simulink model "data_collection"  (R2024a)
settings: Solver=FixedStepAuto  StartTime=0.0  StopTime=inf  FixedStep=0.01  RelTol=1e-3
values from neighbouring files (symbols this model uses):
  omega_max = Simulink.Parameter(425.47)    [katech_automation.m]
  wind_type_toggle = 2    [katech_automation.m]    (also in katech_automation_HILS.m)
  window_size_ = Simulink.Parameter(100)    [katech_automation.m]    (also in katech_automation_HILS.m)
undefined symbols (not defined in the file or in its folder): rad, s, X, Y, Z
libraries: robotlib x28, simulink x14, aerolibconvert2 x2, sharedtransform x1, simulink_extras x1, eeGeneralControl x1
(part 1 of 2)
settings Model: Creator=hmcl  LastModifiedBy=hmcl
settings OptimizationCC: EnhancedBackFolding=on  PassReuseOutputArgsAs=Individual arguments  ZeroExternalMemoryAtStartup=off  ZeroInternalMemoryAtStartup=off  MaxStackSize=64  OptimizeBlockOrder=speed  DifferentSizesBufferReuse=on  OptimizationCustomize=off  EfficientTunableParamExpr=on
settings DebuggingCC: ParameterTunabilityLossMsg=error
settings HardwareCC: ProdBitPerPointer=32  ProdBitPerSizeT=32  ProdBitPerPtrDiffT=32  ProdLargestAtomicFloat=None  ProdIntDivRoundTo=Undefined  ProdEndianess=Unspecified  ProdWordSize=32  ProdHWDeviceType=Generic->Unspecified (assume 32-bit Generic)
settings RTWCC: Description=Embedded Coder  SystemTargetFile=ert.tlc  HardwareBoard=Robot Operating System (ROS)  TLCOptions="-aInlineSetEventsForThisBaseRateFcn=TLC_FALSE -aSuppressMultiTaskScheduler=TLC_FALSE  -aRateBasedStepFcn=0"  TemplateMakefile=ert_default_tmf  Toolchain=Catkin  TargetLang=C++  GPUComputeCapability=3.5
settings CodeAppCC: ForceParamTrailComments=on  IgnoreCustomStorageClasses=off  OperatorAnnotations=on  SimulinkDataObjDesc=on  SFDataObjDesc=on  InsertBlockDesc=on

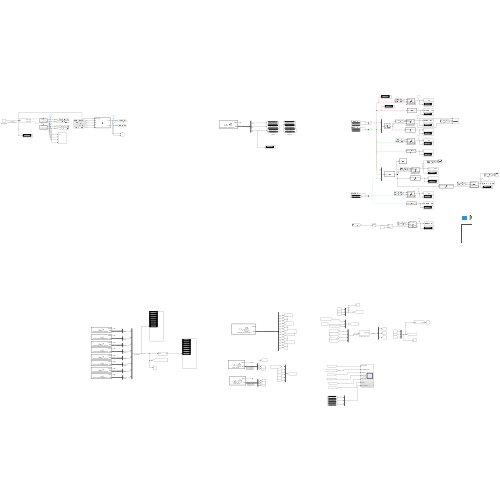
[thumbnail: Simulink's stored preview of the top-level diagram]
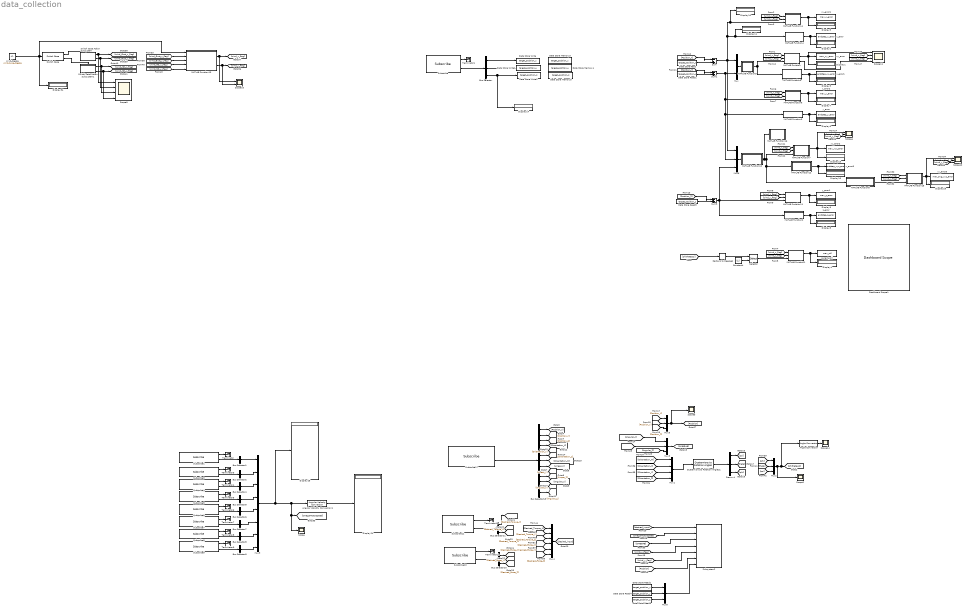
== system data_collection ==
  Angle Conversion : aerolibconvert2/Angle Conversion  IU=rad  OU=deg
  Angular Velocity Conversion1 : aerolibconvert2/Angular Velocity Conversion  IU=rad/s  OU=rpm
  Bus Selector : BusSelector  OutputSignals=Pose.Position.X,Pose.Position.Y,Pose.Position.Z
  Bus Selector{1..2,4..9} (8 alike) : BusSelector  OutputSignals=Data
  Bus Selector10 : BusSelector  OutputSignals=X,Y,Z
  Bus Selector11 : BusSelector  OutputSignals=X,Y,Z
  Bus Selector18 : BusSelector  OutputSignals=Pose.Pose.Position.X,Pose.Pose.Position.Y,Pose.Pose.Position.Z,Pose.Pose.Orientation.X,Pose.Pose.Orientation.Y,Pose.Pose.Orientation.Z,Pose.Pose.Orientation.W,Twist.Twist.Linear.X,Twist.Twist.Linear.Y,Twist.Twist.Linear.Z,Twist.Twist.Angular.X,Twist.Twist.Angular.Y,Twist.Twist.Angular.Z
  Constant4 : Constant  Value=[1]
  Dashboard Scope1 : DashboardScope
  Data Store Memory3 : DataStoreMemory  DataStoreName=target_position_x  ReadBeforeWriteMsg=warning  WriteAfterWriteMsg=warning  WriteAfterReadMsg=warning  ShowAdditionalParam=off
  Data Store Memory4 : DataStoreMemory  DataStoreName=target_position_y  ReadBeforeWriteMsg=warning  WriteAfterWriteMsg=warning  WriteAfterReadMsg=warning  ShowAdditionalParam=off
  Data Store Memory5 : DataStoreMemory  DataStoreName=target_position_z  ReadBeforeWriteMsg=warning  WriteAfterWriteMsg=warning  WriteAfterReadMsg=warning  ShowAdditionalParam=off
  Data Store Read : DataStoreRead  DataStoreName=target_position_x  IndexOptions=Index vector (dialog)  Indices=1  OutputSizes=1
  Data Store Read1 : DataStoreRead  DataStoreName=target_position_y  IndexOptions=Index vector (dialog)  Indices=1  OutputSizes=1
  Data Store Read2 : DataStoreRead  DataStoreName=target_position_x  IndexOptions=Index vector (dialog)  Indices=1  OutputSizes=1
  Data Store Read3 : DataStoreRead  DataStoreName=target_position_z  IndexOptions=Index vector (dialog)  Indices=1  OutputSizes=1
  Data Store Read4 : DataStoreRead  DataStoreName=target_position_y  IndexOptions=Index vector (dialog)  Indices=1  OutputSizes=1
  Data Store Read5 : DataStoreRead  DataStoreName=target_position_z  IndexOptions=Index vector (dialog)  Indices=1  OutputSizes=1
  Data Store Write : DataStoreWrite  DataStoreName=target_position_x  IndexOptions=Index vector (dialog)  Indices=1  OutputSizes=1
  Data Store Write1 : DataStoreWrite  DataStoreName=target_position_y  IndexOptions=Index vector (dialog)  Indices=1  OutputSizes=1
  Data Store Write2 : DataStoreWrite  DataStoreName=target_position_z  IndexOptions=Index vector (dialog)  Indices=1  OutputSizes=1
  Demux4 : Demux  Outputs=3
  Display{1..11,14..16,24..25,29,34} (18 alike) : Display
  MATLAB Function : MATLAB Function  TreatAsAtomicUnit=on
  MATLAB Function1 : MATLAB Function  TreatAsAtomicUnit=on
  MATLAB Function10 : MATLAB Function  TreatAsAtomicUnit=on
  MATLAB Function11 : MATLAB Function  TreatAsAtomicUnit=on
  MATLAB Function12 : MATLAB Function  TreatAsAtomicUnit=on
  MATLAB Function13 : MATLAB Function  TreatAsAtomicUnit=on
  MATLAB Function14 : MATLAB Function  TreatAsAtomicUnit=on
  MATLAB Function15 : MATLAB Function  TreatAsAtomicUnit=on
  MATLAB Function16 : MATLAB Function  TreatAsAtomicUnit=on
  MATLAB Function2 : MATLAB Function  TreatAsAtomicUnit=on
  MATLAB Function3 : MATLAB Function  TreatAsAtomicUnit=on
  MATLAB Function4 : MATLAB Function  TreatAsAtomicUnit=on
  MATLAB Function5 : MATLAB Function  TreatAsAtomicUnit=on
  MATLAB Function6 : MATLAB Function  TreatAsAtomicUnit=on
  MATLAB Function7 : MATLAB Function  TreatAsAtomicUnit=on
  MATLAB Function8 : MATLAB Function  InitFcn=|  TreatAsAtomicUnit=on
      | % 이 코드는 시뮬레이션이 시작되기 직전에 실행됩니다.
      | 
      | % 1. 'window_size_'가 Base Workspace에 '존재하지 않는지' 확인합니다.
      | if ~evalin('base', 'exist(''window_size_'', ''var'')')
      | 
      |     % 존재하지 않으면 (스크립트에서 설정을 잊었으면), 기본값으로 생성합니다.
      |     disp('[InitFcn] "window_size_"를 찾을 수 없습니다. 기본값(100)으로 설정합니다.');
      |     window_size_ = Simulink.Parameter(100);
      | 
      |     % Simulink가 찾을 수 있도록 Base Workspace에 변수를 할당합니다.
      |     assignin('base', 'window_size_', window_size_);
      | end
      | 
      | 
      | try
      |     % 현재 실행 중인 Simulink 모델(.slx)이 저장된 폴더의 '전체 경로'를 찾습니다.
      |     current_model_folder = fileparts(which(bdroot));
      |     
      |     % 'octo_model' 폴더의 '전체 경로'를 생성합니다.
      |     % (Simulink 파일과 'octo_model' 폴더가 같은 디렉터리에 있다고 가정)
      |     path_to_add = fullfile(current_model_folder, 'octo_model');
      |     
      |     % MATLAB 경로에 해당 폴더가 없으면 추가합니다.
      |     if ~contains(path, path_to_add)
      |         disp(['[InitFcn] 함수 경로를 추가합니다: ' path_to_add]);
      |         addpath(path_to_add);
      |     else
      |         disp('[InitFcn] 함수 경로가 이미 설정되어 있습니다.');
      |     end
      | catch ME_path
      |     warndlg(['[InitFcn] 경로 설정 중 심각한 오류 발생: ' ME_path.message], 'InitFcn Error');
      |     return; % 경로 설정 실패 시 중단
      | end
  MATLAB Function9 : MATLAB Function  TreatAsAtomicUnit=on
  Mux : Mux  Inputs=2
  Mux1 : Mux
  Mux{2..3,5..6,8} (5 alike) : Mux  Inputs=3
  Mux4 : Mux  Inputs=6
  Mux9 : Mux  Inputs=8
  Quaternions to Rotation Angles1 : sharedtransform/Quaternions to Rotation Angles  rotationOrder=ZYX  aMode=aMode
  Radians to Degrees : simulink_extras/Transformations/Radians to Degrees
  Scope{,2..3,14} (4 alike) : Scope
  Scope10 : Scope  NumInputPorts=2
  Scope11 : Scope  NumInputPorts=4
  Scope12 : Scope  NumInputPorts=3
  Scope4 : Scope  NumInputPorts=3
  Scope9 : Scope  NumInputPorts=4
  Selector : Selector  InputPortWidth=3  IndexOptions=Index vector (port)  Indices=[1 3]  OutputSizes=1
  Subscribe : robotlib/Subscribe  topicSource=Select from ROS network  topic=/mavros/setpoint_position/local  messageType=geometry_msgs/PoseStamped  SampleTime=-1  legacyBusStruct=off  messageQueueLength=1
  Subscribe1 : robotlib/Subscribe  topicSource=Select from ROS network  topic=/my/octocopter3/motor_speed/0  messageType=std_msgs/Float64  SampleTime=-1  legacyBusStruct=off  messageQueueLength=1
  Subscribe10 : robotlib/Subscribe  topicSource=Select from ROS network  topic=/thrust_vector  messageType=geometry_msgs/Vector3  SampleTime=-1  legacyBusStruct=off  messageQueueLength=1
  Subscribe11 : robotlib/Subscribe  topicSource=Select from ROS network  topic=/torque_vector  messageType=geometry_msgs/Vector3  SampleTime=-1  legacyBusStruct=off  messageQueueLength=1
  Subscribe17 : robotlib/Subscribe  topicSource=Select from ROS network  topic=/mavros/local_position/odom  messageType=nav_msgs/Odometry  SampleTime=-1  legacyBusStruct=off  messageQueueLength=1
  Subscribe3 : robotlib/Subscribe  topicSource=Select from ROS network  topic=/my/octocopter3/motor_speed/1  messageType=std_msgs/Float64  SampleTime=-1  legacyBusStruct=off  messageQueueLength=1
  Subscribe4 : robotlib/Subscribe  topicSource=Select from ROS network  topic=/my/octocopter3/motor_speed/2  messageType=std_msgs/Float64  SampleTime=-1  legacyBusStruct=off  messageQueueLength=1
  Subscribe5 : robotlib/Subscribe  topicSource=Select from ROS network  topic=/my/octocopter3/motor_speed/3  messageType=std_msgs/Float64  SampleTime=-1  legacyBusStruct=off  messageQueueLength=1
  Subscribe6 : robotlib/Subscribe  topicSource=Select from ROS network  topic=/my/octocopter3/motor_speed/4  messageType=std_msgs/Float64  SampleTime=-1  legacyBusStruct=off  messageQueueLength=1
  Subscribe7 : robotlib/Subscribe  topicSource=Select from ROS network  topic=/my/octocopter3/motor_speed/5  messageType=std_msgs/Float64  SampleTime=-1  legacyBusStruct=off  messageQueueLength=1
  Subscribe8 : robotlib/Subscribe  topicSource=Select from ROS network  topic=/my/octocopter3/motor_speed/6  messageType=std_msgs/Float64  SampleTime=-1  legacyBusStruct=off  messageQueueLength=1
  Subscribe9 : robotlib/Subscribe  topicSource=Select from ROS network  topic=/my/octocopter3/motor_speed/7  messageType=std_msgs/Float64  SampleTime=-1  legacyBusStruct=off  messageQueueLength=1
  Subsystem2 : Subsystem
  Sum : Sum  Inputs=|-+
  Sum1 : Sum  Inputs=|-+
  Sum3 : Sum  Inputs=|-+
  Switch Case : SwitchCase  CaseConditions={1,2}  ShowDefaultCase=off
  Switch Case Action Subsystem : Subsystem  TreatAsAtomicUnit=on
  Switch Case Action Subsystem1 : Subsystem  TreatAsAtomicUnit=on
  Terminator{,1,3..11} (11 alike) : Terminator
  current_roll : ToWorkspace  VariableName=max_roll  SampleTime=-1
      settings: Save2DSignal=2-D array (concatenate along first dimension)
  wind_toggle : Constant  InitFcn=|  Value=wind_type_toggle
      | % 이 코드는 시뮬레이션이 시작되기 직전에 실행됩니다.
      | 
      | if ~evalin('base', 'exist(''wind_type_toggle'', ''var'')')
      | 
      |     % 존재하지 않으면 (스크립트에서 설정을 잊었으면), 기본값으로 생성합니다.
      |     disp('[InitFcn] "wind_type_toggle"를 찾을 수 없습니다. 기본값(1, Gust)으로 설정합니다.');
      |     wind_type_toggle = Simulink.Parameter(1);
      | 
      |     % Simulink가 찾을 수 있도록 Base Workspace에 변수를 할당합니다.
      |     assignin('base', 'wind_type_toggle', wind_type_toggle);
      | end
  x_error : ToWorkspace  VariableName=endstep_x_error  SampleTime=-1
      settings: Save2DSignal=2-D array (concatenate along first dimension)
  x_error1 : ToWorkspace  VariableName=endstep_xy_error  SampleTime=-1
      settings: Save2DSignal=2-D array (concatenate along first dimension)
  x_error2 : ToWorkspace  VariableName=max_y_error  SampleTime=-1
      settings: Save2DSignal=2-D array (concatenate along first dimension)
  x_error3 : ToWorkspace  VariableName=endstep_xyz_error  SampleTime=-1
      settings: Save2DSignal=2-D array (concatenate along first dimension)
  xy_error : ToWorkspace  VariableName=max_xy_error  SampleTime=-1
      settings: Save2DSignal=2-D array (concatenate along first dimension)
  xy_error1 : ToWorkspace  VariableName=max_x_error  SampleTime=-1
      settings: Save2DSignal=2-D array (concatenate along first dimension)
  xy_error2 : ToWorkspace  VariableName=max_xyz_error  SampleTime=-1
      settings: Save2DSignal=2-D array (concatenate along first dimension)
  xy_error3 : ToWorkspace  VariableName=max_avg_xyz_error  SampleTime=-1
      settings: Save2DSignal=2-D array (concatenate along first dimension)
  y_error : ToWorkspace  VariableName=endstep_y_error  SampleTime=-1
      settings: Save2DSignal=2-D array (concatenate along first dimension)
  y_error1 : ToWorkspace  VariableName=max_z_error  SampleTime=-1
      settings: Save2DSignal=2-D array (concatenate along first dimension)
  z_error : ToWorkspace  VariableName=endstep_z_error  SampleTime=-1
      settings: Save2DSignal=2-D array (concatenate along first dimension)
  wires:
  Bus Selector/3 -> Display14/1, Data Store Write2/1  "<Z>"
  Subscribe/1 -> Terminator1/1
  Bus Selector/2 -> Data Store Write1/1  "<Y>"
  Bus Selector/1 -> Data Store Write/1  "<X>"
  MATLAB Function3/1(y) -> Display6/1, y_error/1
  MATLAB Function2/1(y) -> Display8/1, z_error/1
  MATLAB Function14/1(y) -> Display5/1, xy_error1/1
  MATLAB Function6/1(y) -> Display7/1, x_error2/1
  MATLAB Function/1(y) -> Scope11/1, xy_error/1, Display1/1
  MATLAB Function4/1(y) -> x_error/1, Display2/1
  MATLAB Function11/1(y) -> Display9/1, y_error1/1
  MATLAB Function9/1(y) -> x_error1/1, Display3/1
  Data Store Read/1 -> Sum/2
  [wind_x_flag] -> MATLAB Function14/1(wind_x_flag)
  [wind_x_flag] -> MATLAB Function6/1(wind_x_flag)
  Sum3/1 -> MATLAB Function11/3(u), Mux6/3, MATLAB Function2/1(endstep_z_error)
  [wind_y_flag] -> MATLAB Function/2(wind_y_flag)
  [wind_x_flag] -> MATLAB Function/1(wind_x_flag)
  MATLAB Function5/1(y) -> MATLAB Function9/1(endstep_xy_error), MATLAB Function/3(u)
  [wind_x_flag] -> MATLAB Function11/1(wind_x_flag)
  Data Store Read3/1 -> Sum3/2
  [wind_y_flag] -> MATLAB Function6/2(wind_y_flag)
  Mux/1 -> MATLAB Function5/1(xy_error)
  [wind_y_flag] -> MATLAB Function11/2(wind_y_flag)
  Sum/1 -> Mux6/1, MATLAB Function14/3(u), Display10/1, Display11/1, MATLAB Function4/1(endstep_x_error), Mux/1
  Sum1/1 -> MATLAB Function6/3(u), Mux6/2, MATLAB Function3/1(endstep_y_error), Mux/2
  Data Store Read1/1 -> Sum1/2
  [wind_y_flag] -> MATLAB Function14/2(wind_y_flag)
  MATLAB Function1/1(y) -> Display4/1, current_roll/1
  Constant4/1 -> Selector/2
  [phithetapsi] -> Radians to Degrees/1
  Selector/1 -> MATLAB Function1/3(u)
  [wind_x_flag] -> MATLAB Function1/1(wind_x_flag)
  [wind_y_flag] -> MATLAB Function1/2(wind_y_flag)
  Radians to Degrees/1 -> Selector/1
  Subscribe/2 -> Bus Selector/1
  [Orientation_W] -> Mux1/1  "W"
  Demux4/3 -> [phi]
  Demux4/1 -> [psi]
  Demux4/2 -> [theta]
  [Orientation_Y] -> Mux1/3  "Y"
  Quaternions to Rotation Angles1/1 -> Demux4/1  "radian"
  [Orientation_X] -> Mux1/2  "x"
  [Orientation_Z] -> Mux1/4  "z"
  Mux1/1 -> Quaternions to Rotation Angles1/1  "quertanion"
  [phi] -> Mux2/1
  Mux2/1 -> Scope2/1, Angle Conversion/1, [phithetapsi]
  [psi] -> Mux2/3
  [theta] -> Mux2/2
  [Position_X] -> Sum/1
  [Position_Y] -> Sum1/1
  [Position_Z] -> Sum3/1
  [Angular_X] -> Mux3/1
  [Angular_Y] -> Mux3/2
  [Angular_Z] -> Mux3/3
  Mux3/1 -> [OMEGAB]
  [OMEGAB] -> Subsystem2/3(OMEGAB)
  [desired_input] -> Subsystem2/1(desired_input)
  [omegaMotorSpeed] -> Subsystem2/2(omegaMotorSpeed)
  Bus Selector8/1 -> Mux9/7  "<Data>"
  Subscribe1/1 -> Terminator/1
  Subscribe8/2 -> Bus Selector8/1
  Subscribe3/1 -> Terminator3/1
  Subscribe3/2 -> Bus Selector2/1
  Subscribe4/2 -> Bus Selector4/1
  Bus Selector4/1 -> Mux9/3  "<Data>"
  Angular Velocity Conversion1/1 -> Display24/1
  Subscribe6/2 -> Bus Selector6/1
  Subscribe4/1 -> Terminator4/1
  Mux9/1 -> Display25/1, Angular Velocity Conversion1/1, Scope/1, [omegaMotorSpeed]  "motorSpeed"
  Subscribe6/1 -> Terminator6/1
  Subscribe9/2 -> Bus Selector9/1
  Bus Selector6/1 -> Mux9/5  "<Data>"
  Subscribe5/2 -> Bus Selector5/1
  Bus Selector9/1 -> Mux9/8  "<Data>"
  Subscribe5/1 -> Terminator5/1
  Subscribe7/1 -> Terminator7/1
  Bus Selector1/1 -> Mux9/1  "<Data>"
  Subscribe1/2 -> Bus Selector1/1
  Subscribe7/2 -> Bus Selector7/1
  Subscribe9/1 -> Terminator9/1
  Subscribe8/1 -> Terminator8/1
  Bus Selector2/1 -> Mux9/2  "<Data>"
  Bus Selector5/1 -> Mux9/4  "<Data>"
  Bus Selector7/1 -> Mux9/6  "<Data>"
  [Desired_Force_X] -> Mux4/4
  [Desired_Torque_Y] -> Mux4/2
  Bus Selector11/3 -> [Desired_Torque_Z]  "<Z>"
  [Desired_Torque_X] -> Mux4/1
  Subscribe10/1 -> Terminator11/1
  Subscribe11/2 -> Bus Selector11/1  "Desired_Torque_X Desired_Torque_Y Desired_Torque_Z"
  [Desired_Torque_Z] -> Mux4/3
  [Desired_Force_Y] -> Mux4/5
  [Desired_Force_Z] -> Mux4/6
  Subscribe11/1 -> Terminator10/1
  Bus Selector10/3 -> [Desired_Force_Z]  "<Z>"
  Bus Selector10/2 -> [Desired_Force_Y]  "<Y>"
  Subscribe10/2 -> Bus Selector10/1  "Desired_Force_X Desired_Force_Y Desired_Force_Z"
  Bus Selector11/1 -> [Desired_Torque_X]  "<X>"
  Bus Selector11/2 -> [Desired_Torque_Y]  "<Y>"
  Bus Selector10/1 -> [Desired_Force_X]  "<X>"
  Mux4/1 -> [desired_input]
  [wind_x_flag] -> Subsystem2/4(wind_x_flag)
  [wind_y_flag] -> Subsystem2/5(wind_y_flag)
  [Position_X] -> Mux5/1
  [Position_Y] -> Mux5/2
  [Position_Z] -> Mux5/3
  Mux5/1 -> Scope3/1, [Position]
  Mux6/1 -> MATLAB Function10/1(xyz_error)
  [wind_x_flag] -> MATLAB Function7/1(wind_x_flag)
  [wind_y_flag] -> MATLAB Function7/2(wind_y_flag)
  MATLAB Function10/1(y) -> MATLAB Function16/1(u), MATLAB Function7/3(u), MATLAB Function8/1(xyz_error), MATLAB Function12/1(endstep_xyz_error)
  MATLAB Function7/1(y) -> Scope4/1, Display15/1, xy_error2/1
  MATLAB Function12/1(y) -> x_error3/1, Display16/1
  [wind_x_flag] -> Scope4/2
  [wind_y_flag] -> Scope4/3
  Switch Case/1 -> Switch Case Action Subsystem/Action
  Switch Case/2 -> Switch Case Action Subsystem1/Action
  Switch Case Action Subsystem1/1(Out1) -> Scope9/3, [wind_ND_x_flag]
  wind_toggle/1 -> Switch Case/1, MATLAB Function13/1(wind_toggle), Display34/1  "1 : Gust 2 : Normal Distribution"
  Switch Case Action Subsystem/1(Out2) -> Scope9/1, [wind_Gust_x_flag]
  Switch Case Action Subsystem/2(Output) -> Scope9/2, [wind_Gust_y_flag]
  MATLAB Function13/1(x_flag) -> Scope10/1, [wind_x_flag]
  MATLAB Function13/2(y_flag) -> Scope10/2, [wind_y_flag]
  [wind_Gust_y_flag] -> MATLAB Function13/3(a2)
  [wind_Gust_x_flag] -> MATLAB Function13/2(a1)
  [wind_ND_x_flag] -> MATLAB Function13/4(a3)
  [wind_ND_y_flag] -> MATLAB Function13/5(a4)
  Switch Case Action Subsystem1/2(Out2) -> Scope9/4, [wind_ND_y_flag]
  [wind_x_flag] -> Scope11/2
  [wind_y_flag] -> Scope11/3
  MATLAB Function/2(toggle_swtich) -> Scope11/4
  Subscribe17/2 -> Bus Selector18/1
  Bus Selector18/1 -> [Position_X]  "<X>"
  Bus Selector18/2 -> [Position_Y]  "<Y>"
  Bus Selector18/3 -> [Position_Z]  "<Z>"
  Bus Selector18/4 -> [Orientation_X]  "<X>"
  Bus Selector18/5 -> [Orientation_Y]  "<Y>"
  Bus Selector18/6 -> [Orientation_Z]  "<Z>"
  Bus Selector18/7 -> [Orientation_W]  "<W>"
  Bus Selector18/8 -> [Linear_X]  "<X>"
  Bus Selector18/9 -> [Linear_Y]  "<Y>"
  Bus Selector18/10 -> [Linear_Z]  "<Z>"
  Bus Selector18/11 -> [Angular_X]  "<X>"
  Bus Selector18/12 -> [Angular_Y]  "<Y>"
  Bus Selector18/13 -> [Angular_Z]  "<Z>"
  [Position] -> Subsystem2/6(Position)
  MATLAB Function8/1(avg_array_xyz_error) -> MATLAB Function15/3(u)
  [wind_x_flag] -> MATLAB Function15/1(wind_x_flag)
  [wind_y_flag] -> MATLAB Function15/2(wind_y_flag)
  [wind_y_flag] -> Scope12/3
  [wind_x_flag] -> Scope12/2
  MATLAB Function15/1(y) -> Display29/1, Scope12/1, xy_error3/1
  Angle Conversion/1 -> Scope14/1
  Data Store Read5/1 -> Mux8/3
  Data Store Read4/1 -> Mux8/2
  Data Store Read2/1 -> Mux8/1
  Mux8/1 -> Subsystem2/7(Target Position)

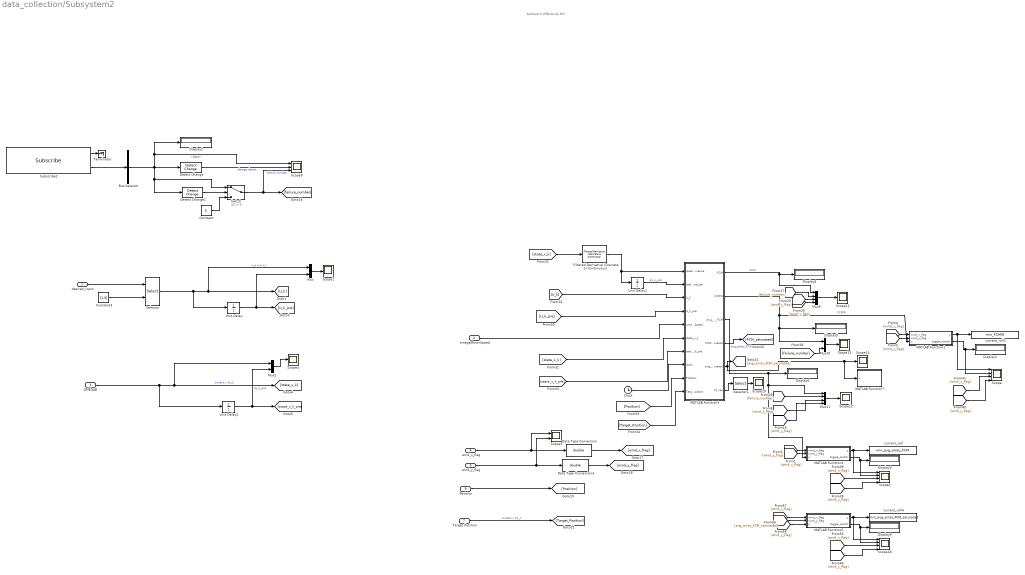
== system data_collection/Subsystem2 ==
  note: backward difference fcm
  desired_input : Inport
  omegaMotorSpeed : Inport  Port=2
  OMEGAB : Inport  Port=3
  wind_x_flag : Inport  Port=4
  wind_y_flag : Inport  Port=5
  Position : Inport  Port=6
  Target Position : Inport  Port=7
  Bus Selector : BusSelector  OutputSignals=Data
  Clock : Clock
  Constant : Constant  Value=0
  Constant4 : Constant  Value=[1:3]
  Data Type Conversion : DataTypeConversion  OutDataTypeStr=double  SaturateOnIntegerOverflow=off  RndMeth=Floor
  Data Type Conversion1 : DataTypeConversion  OutDataTypeStr=double  SaturateOnIntegerOverflow=off  RndMeth=Floor
  Detect Change : simulink/Logic and Bit Operations/Detect Change  vinit=0  OutDataTypeStr=boolean
  Detect Change1 : simulink/Logic and Bit Operations/Detect Change  vinit=0  OutDataTypeStr=boolean
  Display{1..6,9} (7 alike) : Display
  Filtered Derivative (Discrete or Continuous) : eeGeneralControl/Filtered Derivative (Discrete or Continuous)  K=1  T=0.1  B=inf  A=-inf  minRatio=10  init_option=Inherited from block input  x0=0  Ts=-1
      settings: LibrarySourceBlock=|
      | ee_sl_lib/General Control/Filtered Derivative
      | (Discrete or Continuous)
  MATLAB Function2 : MATLAB Function  TreatAsAtomicUnit=on
  MATLAB Function3 : MATLAB Function  InitFcn=|  TreatAsAtomicUnit=on
      | % 이 코드는 시뮬레이션이 시작되기 직전에 실행됩니다.
      | 
      | % 1. 'window_size_'가 Base Workspace에 '존재하지 않는지' 확인합니다.
      | if ~evalin('base', 'exist(''window_size_'', ''var'')')
      | 
      |     % 존재하지 않으면 (스크립트에서 설정을 잊었으면), 기본값으로 생성합니다.
      |     disp('[InitFcn] "window_size_"를 찾을 수 없습니다. 기본값(100)으로 설정합니다.');
      |     window_size_ = Simulink.Parameter(100);
      | 
      |     % Simulink가 찾을 수 있도록 Base Workspace에 변수를 할당합니다.
      |     assignin('base', 'window_size_', window_size_);
      | end
      | 
      | % 2. 'omega_max'가 Base Workspace에 '존재하지 않는지' 확인합니다.
      | if ~evalin('base', 'exist(''omega_max'', ''var'')')
      | 
      |     % 존재하지 않으면, 기본값으로 생성합니다.
      |     disp('[InitFcn] "omega_max"를 찾을 수 없습니다. 기본값(425.47)으로 설정합니다.');
      |     omega_max = Simulink.Parameter(425.47);
      | 
      |     % Base Workspace에 변수를 할당합니다.
      |     assignin('base', 'omega_max', omega_max);
      | end
      | 
      | 
      | try
      |     % 현재 실행 중인 Simulink 모델(.slx)이 저장된 폴더의 '전체 경로'를 찾습니다.
      |     current_model_folder = fileparts(which(bdroot));
      |     
      |     % 'octo_model' 폴더의 '전체 경로'를 생성합니다.
      |     % (Simulink 파일과 'octo_model' 폴더가 같은 디렉터리에 있다고 가정)
      |     path_to_add = fullfile(current_model_folder, 'octo_model');
      |     
      |     % MATLAB 경로에 해당 폴더가 없으면 추가합니다.
      |     if ~contains(path, path_to_add)
      |         disp(['[InitFcn] 함수 경로를 추가합니다: ' path_to_add]);
      |         addpath(path_to_add);
      |     else
      |         disp('[InitFcn] 함수 경로가 이미 설정되어 있습니다.');
      |     end
      | catch ME_path
      |     warndlg(['[InitFcn] 경로 설정 중 심각한 오류 발생: ' ME_path.message], 'InitFcn Error');
      |     return; % 경로 설정 실패 시 중단
      | end
      | 
      | 
      | % --- 2. [필수] 모델 파라미터 스크립트 실행 ---
      | try
      |     % 'octo_model' 폴더 내의 스크립트 '전체 경로'를 만듭니다.
      |     script_to_run = fullfile(path_to_add, 'octocopter_model_for_agressive.m');
      |     
      |     % ★중요★: 스크립트 파일이 실제로 존재하는지 확인
      |     if isfile(script_to_run)
      |         disp(['[InitFcn] 모델 스크립트 실행: ' script_to_run]);
      |         % 'run' 명령어는 '전체 경로'로 실행해야 안전합니다.
      |         run(script_to_run);
      |     else
      |         % 파일이 없으면 시뮬레이션 중지
      |         error_msg = ['[InitFcn] FATAL: 모델 스크립트 파일을 찾을 수 없습니다: ' script_to_run];
      |         disp(error_msg);
      |         warndlg(error_msg, 'InitFcn Error');
      |         return; % 스크립트 없음
      |     end
      | catch ME_run
      |     disp('[InitFcn] 모델 스크립트 실행 중 오류 발생:');
      |     disp(ME_run.message);
      |     warndlg(['모델 스크립트(' script_to_run ') 실행에 실패했습니다: ' ME_run.message], 'InitFcn Error');
      |     return; % 스크립트 실행 실패
      | end
  MATLAB Function4 : MATLAB Function  TreatAsAtomicUnit=on
  MATLAB Function5 : MATLAB Function  TreatAsAtomicUnit=on
  MATLAB Function7 : MATLAB Function  TreatAsAtomicUnit=on
  Mux : Mux  Inputs=2
  Mux10 : Mux  Inputs=2
  Mux11 : Mux
  Mux2 : Mux  Inputs=2
  Mux9 : Mux
  Scope : Scope  NumInputPorts=4
  Scope{1,4,11..14,19} (7 alike) : Scope
  Scope18 : Scope  NumInputPorts=4
  Scope2 : Scope  NumInputPorts=4
  Scope3 : Scope  NumInputPorts=2
  Scope9 : Scope  NumInputPorts=3
  Selector : Selector  InputPortWidth=6  IndexOptions=Index vector (port)  Indices=[1 3]  OutputSizes=1
  Selector1 : Selector  InputPortWidth=9  IndexOptions=Index vector (dialog)  Indices=[1 5 9]  OutputSizes=1
  Subscribe2 : robotlib/Subscribe  topicSource=Select from ROS network  topic=/mavros/keyboard_command/failure_number  messageType=std_msgs/Float32  SampleTime=-1  legacyBusStruct=off  messageQueueLength=1
  Switch : Switch  Criteria=u2 > Threshold  SaturateOnIntegerOverflow=off  InputSameDT=off
  Terminator : Terminator
  Unit Delay : UnitDelay  SampleTime=-1  HasFrameUpgradeWarning=on
  Unit Delay1 : UnitDelay  SampleTime=-1  HasFrameUpgradeWarning=on
  Unit Delay2 : UnitDelay  SampleTime=-1  HasFrameUpgradeWarning=on
  current_roll : ToWorkspace  VariableName=min_avg_array_FCM  SampleTime=-1
      settings: Save2DSignal=2-D array (concatenate along first dimension)
  current_roll1 : ToWorkspace  VariableName=min_FCMW  SampleTime=-1
      settings: Save2DSignal=2-D array (concatenate along first dimension)
  current_roll4 : ToWorkspace  VariableName=min_avg_array_FCM_saturated  SampleTime=-1
      settings: Save2DSignal=2-D array (concatenate along first dimension)
  wires:
  desired_input/1 -> Selector/1
  Unit Delay/1 -> Mux/2, [U_k_pre]
  OMEGAB/1 -> Mux2/1, [state_x_k], Unit Delay1/1  "current x dx_k"
  Unit Delay1/1 -> Mux2/2, [state_x_k_pre]  "dx_k_pre"
  Constant4/1 -> Selector/2
  Selector/1 -> Mux/1, [U_k], Unit Delay/1  "u_p u_q u_r"
  Mux/1 -> Scope1/1
  Mux2/1 -> Scope4/1
  Subscribe2/1 -> Terminator/1
  Subscribe2/2 -> Bus Selector/1
  Bus Selector/1 -> Switch/1, Detect Change1/1, Scope9/1, Display2/1, Detect Change/1  "<Data>"
  Detect Change/1 -> Scope9/2  "change detect"
  Detect Change1/1 -> Switch/2
  Switch/1 -> [failure_number], Scope9/3  "failure number"
  Constant/1 -> Switch/3
  [failure_number] -> Mux9/2
  Mux11/1 -> Scope12/1
  MATLAB Function3/2(FCMW) -> Mux10/1, Display5/1, MATLAB Function2/3(u)  "FCMW"
  [state_x_k] -> Filtered Derivative (Discrete or Continuous)/1
  [U_k_pre] -> MATLAB Function3/4(U_k_pre)
  Mux10/1 -> Scope13/1
  [state_x_k] -> MATLAB Function3/6(state_x_k)
  [failure_number] -> Mux10/2
  Mux9/1 -> Scope11/1
  MATLAB Function3/3(avg_array_FCM) -> MATLAB Function4/3(u), Mux11/1, Display6/1  "avg_array_FCM"
  [failure_number] -> Mux11/2
  MATLAB Function3/1(FCM) -> Mux9/1, Display4/1  "FCM"
  [U_k] -> MATLAB Function3/3(U_k)
  omegaMotorSpeed/1 -> MATLAB Function3/5(omegaMotorSpeed)
  [state_x_k_pre] -> MATLAB Function3/7(state_x_k_pre)
  MATLAB Function4/1(y) -> Scope2/1, current_roll/1
  wind_x_flag/1 -> Data Type Conversion/1, Scope3/1
  [wind_x_flag] -> MATLAB Function4/1(wind_x_flag)
  wind_y_flag/1 -> Data Type Conversion1/1, Scope3/2
  [wind_y_flag] -> MATLAB Function4/2(wind_y_flag)
  [wind_x_flag] -> MATLAB Function2/1(wind_x_flag)
  MATLAB Function2/1(y) -> Scope/1, current_roll1/1
  [wind_y_flag] -> MATLAB Function2/2(wind_y_flag)
  MATLAB Function2/2(toggle_swtich) -> Scope/2, Display1/1
  MATLAB Function4/2(toggle_swtich) -> Scope2/2, Display3/1
  Filtered Derivative (Discrete or Continuous)/1 -> Unit Delay2/1, MATLAB Function3/1(state_derivative)
  [wind_x_flag] -> Mux11/3
  [wind_y_flag] -> Mux11/4
  [wind_x_flag] -> Mux9/3
  [wind_y_flag] -> Mux9/4
  [wind_x_flag] -> Scope2/3
  [wind_y_flag] -> Scope2/4
  [wind_x_flag] -> Scope/3
  [wind_y_flag] -> Scope/4
  Data Type Conversion/1 -> [wind_x_flag]
  Data Type Conversion1/1 -> [wind_y_flag]
  Clock/1 -> MATLAB Function3/8(clock)
  Position/1 -> [Position]
  [Position] -> MATLAB Function3/9(Position)
  MATLAB Function3/4(FCM_saturated) -> [FCM_saturated]
  MATLAB Function3/5(avg_array_FCM_saturated) -> [avg_array_FCM_saturated], Scope14/1, MATLAB Function7/1(u)
  [wind_x_flag] -> Scope18/3
  MATLAB Function5/2(toggle_swtich) -> Scope18/2, Display9/1
  [wind_y_flag] -> Scope18/4
  MATLAB Function5/1(y) -> Scope18/1, current_roll4/1
  [avg_array_FCM_saturated] -> MATLAB Function5/3(u)
  [wind_x_flag] -> MATLAB Function5/1(wind_x_flag)
  [wind_y_flag] -> MATLAB Function5/2(wind_y_flag)
  MATLAB Function3/6(M_vec) -> Selector1/1
  Selector1/1 -> Scope19/1
  Unit Delay2/1 -> MATLAB Function3/2(state_derivative_pre)  "dx_k_pre"
  Target Position/1 -> [Target_Position]  "current x dx_k"
  [Target_Position] -> MATLAB Function3/10(Target_Position)

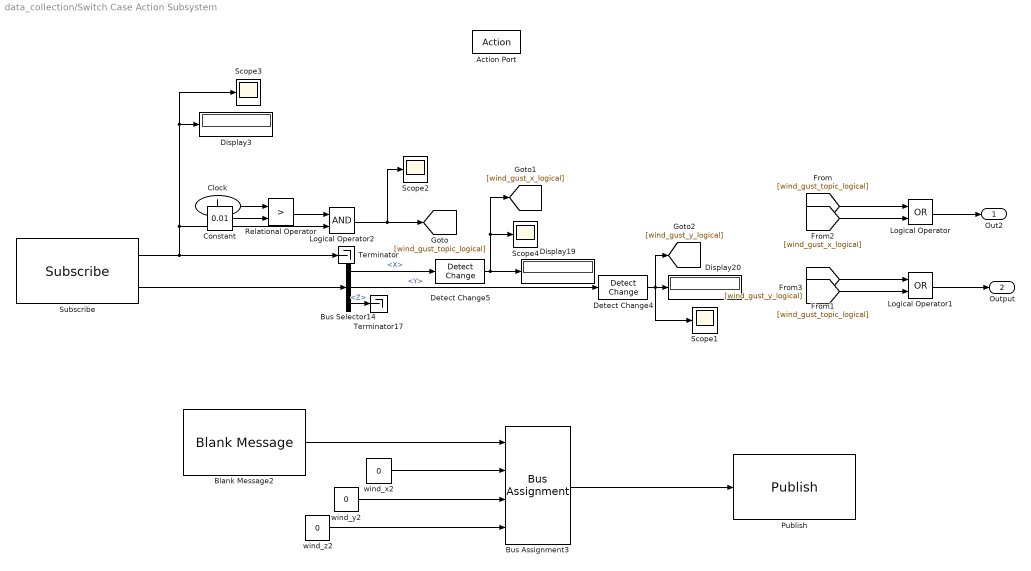
== system data_collection/Switch Case Action Subsystem ==
  Action Port : ActionPort  ActionPortLabel=case [ 1 ]:
  Blank Message2 : robotlib/Blank Message  messageClass=Message  entityType=geometry_msgs/Vector3  messageType=geometry_msgs/Vector3  SampleTime=inf  legacyBusStruct=off
  Bus Assignment3 : BusAssignment  AssignedSignals=X,Y,Z
  Bus Selector14 : BusSelector  OutputSignals=X,Y,Z
  Clock : Clock
  Constant : Constant  Value=0.01
  Detect Change4 : simulink/Logic and Bit Operations/Detect Change  vinit=0  OutDataTypeStr=boolean
  Detect Change5 : simulink/Logic and Bit Operations/Detect Change  vinit=0  OutDataTypeStr=boolean
  Display19 : Display
  Display20 : Display
  Display3 : Display
  Logical Operator : Logic  Operator=OR  AllPortsSameDT=off  OutDataTypeStr=boolean
  Logical Operator1 : Logic  Operator=OR  AllPortsSameDT=off  OutDataTypeStr=boolean
  Logical Operator2 : Logic  AllPortsSameDT=off  OutDataTypeStr=boolean
  Publish : robotlib/Publish  topicSource=Select from ROS network  topic=/wind_gust_pub  messageType=geometry_msgs/Vector3  legacyBusStruct=off  messageQueueLength=1
  Relational Operator : RelationalOperator  Operator=>  OutDataTypeStr=boolean  RndMeth=Simplest  InputSameDT=off
  Scope{1..4} (4 alike) : Scope
  Subscribe : robotlib/Subscribe  topicSource=Select from ROS network  topic=/wind_gust_pub  messageType=geometry_msgs/Vector3  SampleTime=-1  legacyBusStruct=off  messageQueueLength=1
  Terminator : Terminator
  Terminator17 : Terminator
  wind_x2 : Constant  Value=0
  wind_y2 : Constant  Value=0
  wind_z2 : Constant  Value=0
  Out2 : Outport
  Output : Outport  Port=2
  wires:
  Bus Assignment3/1 -> Publish/1
  Blank Message2/1 -> Bus Assignment3/1
  Bus Selector14/3 -> Terminator17/1  "<Z>"
  Detect Change5/1 -> Scope4/1, [wind_gust_x_logical], Display19/1
  wind_x2/1 -> Bus Assignment3/2
  Subscribe/2 -> Bus Selector14/1
  Detect Change4/1 -> [wind_gust_y_logical], Scope1/1, Display20/1
  Bus Selector14/2 -> Detect Change4/1  "<Y>"
  wind_y2/1 -> Bus Assignment3/3
  Subscribe/1 -> Terminator/1, Scope3/1, Display3/1, Logical Operator2/2
  wind_z2/1 -> Bus Assignment3/4
  Bus Selector14/1 -> Detect Change5/1  "<X>"
  Logical Operator/1 -> Out2/1
  Logical Operator1/1 -> Output/1
  [wind_gust_topic_logical] -> Logical Operator/1
  [wind_gust_topic_logical] -> Logical Operator1/1
  [wind_gust_x_logical] -> Logical Operator/2
  [wind_gust_y_logical] -> Logical Operator1/2
  Clock/1 -> Relational Operator/1
  Constant/1 -> Relational Operator/2
  Relational Operator/1 -> Logical Operator2/1
  Logical Operator2/1 -> Scope2/1, [wind_gust_topic_logical]

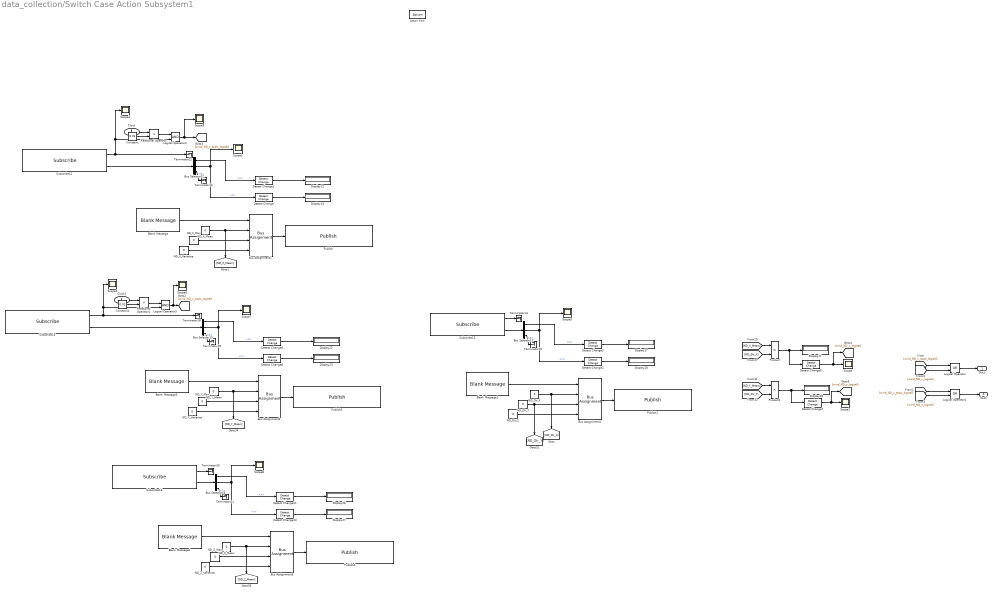
== system data_collection/Switch Case Action Subsystem1 ==
  Action Port : ActionPort  ActionPortLabel=case [ 2 ]:
  Blank Message{,1,3..4} (4 alike) : robotlib/Blank Message  messageClass=Message  entityType=geometry_msgs/Vector3  messageType=geometry_msgs/Vector3  SampleTime=inf  legacyBusStruct=off
  Bus Assignment{1..2,4..5} (4 alike) : BusAssignment  AssignedSignals=X,Y,Z
  Bus Selector{12..13,15..16} (4 alike) : BusSelector  OutputSignals=X,Y,Z
  Clock : Clock
  Clock1 : Clock
  Constant : Constant  Value=0.01
  Constant1 : Constant  Value=0.01
  Detect Change{,1..3,6..11} (10 alike) : simulink/Logic and Bit Operations/Detect Change  vinit=0  OutDataTypeStr=boolean
  Display{12..13,17..18,21..23,26..28} (10 alike) : Display
  Logical Operator : Logic  Operator=OR  AllPortsSameDT=off  OutDataTypeStr=boolean
  Logical Operator1 : Logic  Operator=OR  AllPortsSameDT=off  OutDataTypeStr=boolean
  Logical Operator2 : Logic  AllPortsSameDT=off  OutDataTypeStr=boolean
  Logical Operator3 : Logic  AllPortsSameDT=off  OutDataTypeStr=boolean
  ND_Dir_X : Constant  Value=0
  ND_Dir_Y : Constant  Value=0
  ND_Dir_Z : Constant  Value=0
  ND_X_Max : Constant  Value=0
  ND_X_Mean : Constant  Value=0
  ND_X_Variance : Constant  Value=0
  ND_Y_Max : Constant  Value=0
  ND_Y_Mean : Constant  Value=0
  ND_Y_Variance : Constant  Value=0
  ND_Z_Max : Constant  Value=0
  ND_Z_Mean : Constant  Value=0
  ND_Z_Variance : Constant  Value=0
  Product : Product
  Product1 : Product
  Publish : robotlib/Publish  topicSource=Select from ROS network  topic=/wind_normal_distribution_Mean_Max_Variance_X_pub  messageType=geometry_msgs/Vector3  legacyBusStruct=off  messageQueueLength=1
  Publish1 : robotlib/Publish  topicSource=Select from ROS network  topic=/wind_normal_distribution_XYZ_Direction_pub  messageType=geometry_msgs/Vector3  legacyBusStruct=off  messageQueueLength=1
  Publish3 : robotlib/Publish  topicSource=Select from ROS network  topic=/wind_normal_distribution_Mean_Max_Variance_Y_pub  messageType=geometry_msgs/Vector3  legacyBusStruct=off  messageQueueLength=1
  Publish4 : robotlib/Publish  topicSource=Select from ROS network  topic=/wind_normal_distribution_Mean_Max_Variance_Z_pub  messageType=geometry_msgs/Vector3  legacyBusStruct=off  messageQueueLength=1
  Relational Operator : RelationalOperator  Operator=>  OutDataTypeStr=boolean  RndMeth=Simplest  InputSameDT=off
  Relational Operator1 : RelationalOperator  Operator=>  OutDataTypeStr=boolean  RndMeth=Simplest  InputSameDT=off
  Scope{,1..9} (10 alike) : Scope
  Subscribe12 : robotlib/Subscribe  topicSource=Select from ROS network  topic=/wind_normal_distribution_Mean_Max_Variance_X_pub  messageType=geometry_msgs/Vector3  SampleTime=-1  legacyBusStruct=off  messageQueueLength=1
  Subscribe13 : robotlib/Subscribe  topicSource=Select from ROS network  topic=/wind_normal_distribution_XYZ_Direction_pub  messageType=geometry_msgs/Vector3  SampleTime=-1  legacyBusStruct=off  messageQueueLength=1
  Subscribe15 : robotlib/Subscribe  topicSource=Select from ROS network  topic=/wind_normal_distribution_Mean_Max_Variance_Y_pub  messageType=geometry_msgs/Vector3  SampleTime=-1  legacyBusStruct=off  messageQueueLength=1
  Subscribe16 : robotlib/Subscribe  topicSource=Select from ROS network  topic=/wind_normal_distribution_Mean_Max_Variance_Z_pub  messageType=geometry_msgs/Vector3  SampleTime=-1  legacyBusStruct=off  messageQueueLength=1
  Terminator{12..15,18..21} (8 alike) : Terminator
  Out1 : Outport
  Out2 : Outport  Port=2
  wires:
  Bus Selector15/1 -> Detect Change9/1  "<X>"
  Subscribe16/1 -> Terminator20/1
  Bus Selector13/1 -> Detect Change3/1  "<X>"
  Detect Change1/1 -> Display12/1
  Subscribe16/2 -> Bus Selector16/1
  Bus Selector15/3 -> Terminator19/1  "<Z>"
  Subscribe12/1 -> Terminator12/1, Scope3/1, Logical Operator2/2
  Subscribe13/1 -> Terminator14/1
  Subscribe13/2 -> Bus Selector13/1
  ND_Dir_Y/1 -> Bus Assignment2/3, [ND_Dir_Y]
  Detect Change2/1 -> Display18/1
  Bus Selector16/1 -> Detect Change11/1  "<X>"
  ND_Y_Max/1 -> Bus Assignment4/3
  Product/1 -> Detect Change6/1, Display21/1
  ND_Y_Mean/1 -> Bus Assignment4/2, [ND_Y_Mean]
  Product1/1 -> Display28/1, Detect Change7/1
  Bus Assignment2/1 -> Publish1/1
  ND_Z_Max/1 -> Bus Assignment5/3
  Detect Change8/1 -> Display23/1
  Subscribe12/2 -> Bus Selector12/1
  [ND_X_Mean] -> Product/1
  Bus Selector15/2 -> Detect Change8/1, Scope7/1  "<Y>"
  ND_X_Max/1 -> Bus Assignment1/3
  Bus Assignment4/1 -> Publish3/1
  ND_X_Mean/1 -> Bus Assignment1/2, [ND_X_Mean]
  Detect Change10/1 -> Display27/1
  ND_Dir_X/1 -> Bus Assignment2/2, [ND_Dir_X]
  Subscribe15/1 -> Scope4/1, Logical Operator3/2, Terminator18/1
  ND_Z_Variance/1 -> Bus Assignment5/4
  [ND_Y_Mean] -> Product1/1
  Bus Selector12/3 -> Terminator13/1  "<Z>"
  ND_Y_Variance/1 -> Bus Assignment4/4
  Bus Selector16/2 -> Detect Change10/1, Scope8/1  "<Y>"
  [ND_Dir_X] -> Product/2
  Bus Selector12/2 -> Detect Change/1, Scope1/1  "<Y>"
  ND_Z_Mean/1 -> [ND_Z_Mean], Bus Assignment5/2
  Subscribe15/2 -> Bus Selector15/1
  [ND_Dir_Y] -> Product1/2
  Detect Change9/1 -> Display22/1
  Bus Selector13/3 -> Terminator15/1  "<Z>"
  Detect Change11/1 -> Display26/1
  ND_X_Variance/1 -> Bus Assignment1/4
  Bus Selector16/3 -> Terminator21/1  "<Z>"
  Bus Selector13/2 -> Detect Change2/1, Scope5/1  "<Y>"
  Blank Message/1 -> Bus Assignment1/1
  Blank Message3/1 -> Bus Assignment4/1
  Bus Selector12/1 -> Detect Change1/1  "<X>"
  ND_Dir_Z/1 -> Bus Assignment2/4
  Detect Change3/1 -> Display17/1
  Blank Message4/1 -> Bus Assignment5/1
  Blank Message1/1 -> Bus Assignment2/1
  Detect Change/1 -> Display13/1
  Bus Assignment5/1 -> Publish4/1
  Bus Assignment1/1 -> Publish/1
  Logical Operator/1 -> Out1/1
  [wind_ND_y_logical] -> Logical Operator1/2
  [wind_ND_y_topic_logical] -> Logical Operator1/1
  Logical Operator1/1 -> Out2/1
  [wind_ND_x_topic_logical] -> Logical Operator/1
  [wind_ND_x_logical] -> Logical Operator/2
  Detect Change6/1 -> [wind_ND_x_logical], Scope/1
  Detect Change7/1 -> [wind_ND_y_logical], Scope2/1
  Constant/1 -> Relational Operator/2
  Clock/1 -> Relational Operator/1
  Relational Operator/1 -> Logical Operator2/1
  Logical Operator2/1 -> Scope9/1, [wind_ND_x_topic_logical]
  Relational Operator1/1 -> Logical Operator3/1
  Clock1/1 -> Relational Operator1/1
  Constant1/1 -> Relational Operator1/2
  Logical Operator3/1 -> Scope6/1, [wind_ND_y_topic_logical]

== matlab function data_collection/Subsystem2/MATLAB Function4 ==
  data: wind_x_flag input; wind_y_flag input; u input; y output; toggle_swtich output
function [y, toggle_swtich] = fcn(wind_x_flag, wind_y_flag, u)
    coder.extrinsic('assignin'); % MATLAB 함수 사용을 알림


    % 이전 값을 저장할 persistent 변수 선언
    persistent prev_u;
    persistent toggle_state;
    persistent prev_flag;

    if isempty(prev_u)
        prev_u = -inf; % 초기 값 설정
    end

    if isempty(toggle_state)
        toggle_state = false; % 초기 토글 상태를 논리형으로 설정
    end

    if isempty(prev_flag)
        prev_flag    = false;
    end

    % 현재 플래그 레벨
    curr_flag = wind_x_flag || wind_y_flag;

    % 상승엣지 검출: 이전=0 & 현재=1
    if curr_flag && ~prev_flag
        toggle_state = ~toggle_state;
    end

    prev_flag = curr_flag;    % 엣지 검출을 위한 상태 갱신

    % 현재 토글 상태를 int32 형으로 변환하여 할당
    toggle_swtich = int32(toggle_state);
    % 현재 토글 상태를 출력
    % fprintf('toggle_state = %d \n', toggle_swtich);

    if toggle_state
        % 현재 값이 이전 값보다 큰지 확인
        if abs(u) > abs(prev_u)
            y = abs(prev_u); % 이전 값을 출력
            
        else
            prev_u = abs(u); % 이전 값을 현재 값으로 업데이트
            y = abs(u); % 현재 값을 출력
        end
        assignin('base', 'min_avg_array_FCM', y); % y 값을 MATLAB 기본 워크스페이스의 min_FCMW 저장
    else
        % 토글 상태가 0일 때
        prev_u = 1;
        y = 1;
    end
end




    % if x_change || y_change
    % 
    %     % 현재 값이 이전 값보다 큰지 확인
    %     if u > prev_u
    %         assignin('base', 'current_roll', u);  % u 값을 MATLAB  워크스페이스(base는 MATLAB의 기본 워크스페이스를 의미)의 current_roll에 저장
    %         prev_u = u; % 이전 값을 현재 값으로 업데이트
    %         y = u; % 현재 값을 출력
    %     else
    %         y = prev_u; % 이전 값을 출력
    %     end
    % else
    %     assignin('base', 'current_roll', u);
    %     y = 0;
    % end

== matlab function data_collection/MATLAB Function9 ==
  data: endstep_xy_error input; y output
function y = fcn(endstep_xy_error)

% z_error 값을 기본 워크스페이스에 저장
assignin('base', 'endstep_xy_error', endstep_xy_error);

% 저장된 값을 반환
y = endstep_xy_error;

end

== matlab function data_collection/Subsystem2/MATLAB Function2 ==
  data: wind_x_flag input; wind_y_flag input; u input; y output; toggle_swtich output
function [y, toggle_swtich] = fcn(wind_x_flag, wind_y_flag, u)
    coder.extrinsic('assignin'); % MATLAB 함수 사용을 알림


    % 이전 값을 저장할 persistent 변수 선언
    persistent prev_u;
    persistent toggle_state;
    persistent prev_flag;

    if isempty(prev_u)
        prev_u = -inf; % 초기 값 설정
    end

    if isempty(toggle_state)
        toggle_state = false; % 초기 토글 상태를 논리형으로 설정
    end

    if isempty(prev_flag)
        prev_flag    = false;
    end

    % 현재 플래그 레벨
    curr_flag = wind_x_flag || wind_y_flag;

    % 상승엣지 검출: 이전=0 & 현재=1
    if curr_flag && ~prev_flag
        toggle_state = ~toggle_state;
    end

    prev_flag = curr_flag;    % 엣지 검출을 위한 상태 갱신

    % 현재 토글 상태를 int32 형으로 변환하여 할당
    toggle_swtich = int32(toggle_state);
    % 현재 토글 상태를 출력
    % fprintf('toggle_state = %d \n', toggle_swtich);

    if toggle_state
        % 현재 값이 이전 값보다 큰지 확인
        if abs(u) > abs(prev_u)
            y = abs(prev_u); % 이전 값을 출력
            
        else
            prev_u = abs(u); % 이전 값을 현재 값으로 업데이트
            y = abs(u); % 현재 값을 출력
        end
        assignin('base', 'min_FCMW', y); % y 값을 MATLAB 기본 워크스페이스의 min_FCMW 저장
    else
        % 토글 상태가 0일 때
        prev_u = 1;
        y = 1;
    end
end




    % if x_change || y_change
    % 
    %     % 현재 값이 이전 값보다 큰지 확인
    %     if u > prev_u
    %         assignin('base', 'current_roll', u);  % u 값을 MATLAB  워크스페이스(base는 MATLAB의 기본 워크스페이스를 의미)의 current_roll에 저장
    %         prev_u = u; % 이전 값을 현재 값으로 업데이트
    %         y = u; % 현재 값을 출력
    %     else
    %         y = prev_u; % 이전 값을 출력
    %     end
    % else
    %     assignin('base', 'current_roll', u);
    %     y = 0;
    % end

== matlab function data_collection/Subsystem2/MATLAB Function3 ==
  settings: updateMethod=DISCRETE
  data: state_derivative input; state_derivative_pre input; U_k input; U_k_pre input; FCM output; omegaMotorSpeed input; state_x_k input; state_x_k_pre input; FCMW output; avg_array_FCM output; clock input; Position input; Target_Position input; FCM_saturated output; avg_array_FCM_saturated output; M_vec output size=9; window_size_ parameter; omega_max parameter
function [FCM, FCMW, avg_array_FCM, FCM_saturated, avg_array_FCM_saturated,M_vec]  = fcn(state_derivative,state_derivative_pre,U_k,U_k_pre,omegaMotorSpeed,state_x_k,state_x_k_pre,clock, Position, Target_Position, window_size_, omega_max)
%#codegen

% X_k = current
% X_k_pre = previous
disp('clock = ');
disp(clock);

coder.extrinsic('size');
coder.extrinsic('ctrb');
coder.extrinsic('rank');
coder.extrinsic('inv');
coder.extrinsic('sign');
coder.extrinsic('evalin');
coder.extrinsic('diff');
coder.extrinsic('addpath');
% addpath('/home/hmcl/PX4_testbed/gp_matlab/octo_model');

coder.extrinsic('delft_evaluate_jacobians.m');
coder.extrinsic('calculate_FCMW.m');
coder.extrinsic('calculate_FCMW_saturated.m')

% persistent 변수 선언
persistent initialized avg_array_FCM_ avg_array_FCM_saturated_;
persistent M_prev;



if isempty(M_prev)
    M_prev = eye(3);
end


dt = 0.01; % 시간 간격 % 가제보는 dt = 0.004 로 데이터를 전송및 한다
tau = 0.01; % 액추에이터 시간 상수
M = eye(3);
% window_size_ = 100;

delft_df_dx = zeros(length(state_x_k), length(state_x_k));
delft_df_du = zeros(length(state_x_k), length(U_k));
del_umax = zeros(3,1);
del_uc = zeros(3,1);
signMask = zeros(1,8);
refOmega = zeros(8,1);
signError = zeros(1,1);
rank_con = 0;


rotorMapping = [-1 -1 1;
    1 1 1;
    -1 -1 -1;
    -1 1 -1;
    1 -1 -1;
    1 1 -1;
    1 -1 1;
    -1 1 1];

% rotorMapping = rotorMapping *-1; 

% x = state_x_k1(1);
% y = state_x_k1(2);
% z = state_x_k1(3);
% u = state_x_k1(4);
% v = state_x_k1(5);
% w = state_x_k1(6);
% phi = state_x_k1(7);
% theta = state_x_k1(8);
% psi = state_x_k1(9);
p = state_x_k(1);
q = state_x_k(2);
r = state_x_k(3);

u_p = U_k(1);
u_q = U_k(2);
u_r = U_k(3);

x = Position(1);
y = Position(2);
z = Position(3);

target_x = Target_Position(1);
target_y = Target_Position(2);
target_z = Target_Position(3);



% 초기화가 필요할 때만 실행
if isempty(initialized)
    initialized = true; % 초기화 완료 표시
    FCMW = 1;
    avg_array_FCM = 1.0;
    avg_array_FCM_ = 1.0;

    FCMW_saturated = 1;
    avg_array_FCM_saturated = 1.0;
    avg_array_FCM_saturated_ = 1.0;
    disp('initialized. in MATLAB Function3');
    % disp('window_size_ in MATLAB Function3'); disp(window_size_);
end

disp('-----------------');
% 심볼릭 야코비안 행렬 평가
[df_dx_temp, df_du_temp] = delft_evaluate_jacobians(p, q, r, u_p, u_q, u_r);

% 외부 함수로부터 받은 값을 MATLAB 배열로 변환
delft_df_dx = df_dx_temp; %delft_df_dx = A %3by3   %length(X_k1) by length(X_k1)

delft_df_du = df_du_temp; %delft_df_du = B %3by3    %length(X_k1) by length(U_k1)

A = delft_df_dx;
B = delft_df_du;

debug_info = struct(); 
debug_info.clock = clock;
debug_info.A = A;
debug_info.B_initial = B; 

% 상태 및 입력 차이 계산
diffrate = state_x_k - state_x_k_pre;  % dx는 3x1
du = U_k - U_k_pre;  % du는 3x1

diff_ratedot = state_derivative - state_derivative_pre;




% disp('A = ')
% disp(A)
% disp('du = ')
% disp(du)

% dx_dot = df_dx * dx + df_du * du;
%{
state X 가 정확값이라고 했을때 state X를 미분하면 dx_dot 이 나오게 된다.
그리고 식(6)을 보면 dx_dot 을 근사한 식인 A * dx + B * du 가 있다.
만약 근사한식이 너무 정확하면 dx_dot - (A * dx + B * du) 을 했을때 0 이 된다.
즉, 근사한 식이 정확하면 미분한 식(dx_dot) - 근사한식(A * dx + B * du) 이 0이 되야한다.

하지만 근사한식이 당연히 정확할수 없기 때문에 error가 생기는데
이 에러를 보상해주기 위해, 또는 0으로 수렴 시키기 위해서
del_uc를 정의 해준다.
del_uc는 inv(B) *error 이다.

그래서 dx_dot - (A * dx + B * du + del_uc) 식(11)이 나오고 이 식은 0으로 점점 수렴하게 된다.
%}

error = diff_ratedot - A * diffrate;
debug_info.ER = error; % M 계산에 사용되는 error

M = M_prev; 

% corrcoef_result = corrcoef(state_derivative, A * dx + B * du);
corrcoef_result = corrcoef(diff_ratedot, B * du);

disp('error = ')
disp(error);
disp('B * du = ')
disp(B * du);

for i = 1:3
    if ~isnan(corrcoef_result(1,2))
        M(i, i) = max(corrcoef_result(1,2), 0.001); % 최소값 설정
    end
end
debug_info.corrcoef_result = corrcoef_result;                                                 
debug_info.M = M;

% disp('ER = ')
% disp(error)
% disp('M = ');
% disp(M);
M_vec = M(:);

disp('corrcoef_result = ')
disp(corrcoef_result);

% disp('B = ')
% disp(B)

B = B * M;
debug_info.B_updated = B; % M을 곱한 후 B


M_prev = M;

% disp('B = ')
% disp(B)


% disp('A * dx + B * du = ');
% disp(A * diffrate + B * du);

err = error - B * du; %error : 3by1
% disp('error = ');
% disp(err);
debug_info.err_final = err; % del_uc 계산에 사용되는 최종 error

if (abs(err) == 0)
    
    disp('error is zero');
    FCM = 1;
    FCMW = 1;
    FCM_saturated = 1;

    FCMW_saturated = 1;
    avg_array_FCM = avg_array_FCM_;
    avg_array_FCM_saturated = avg_array_FCM_saturated_;
    return

else
    del_uc = (inv(B)) * err; % del_uc는 3x1
debug_info.del_uc_abs = abs(del_uc);


    rotorMapping_T = rotorMapping'; % 이건 필수인듯?



    % error의 부호를 계산
    for i = 1:length(err)

        signError = sign(err(i));

        signMask = signError .* rotorMapping_T(i,:); % sign(error)를 대체
 

        for j = 1:length(signMask)
            if signMask(j) < 0
                refOmega(j) = omega_max; % signMask가 0보다 작으면 omega_max 할당
            else
                refOmega(j) = 0;         % signMask가 0 이상이면 0 할당
            end
        end

   

        % omegaMotorSpeed [rad/s]
        maxDiff = abs(abs(omegaMotorSpeed) - refOmega); %maxDiff  8by1
  

        % Δu_MAX
        del_umax(i,1) = dt * (1/tau) * sum(maxDiff);

    end
        debug_info.del_umax = del_umax;



    controllability_matrix = ctrb(A,B);
    % disp('controllability_matrix = ')
    % disp(controllability_matrix)

    % 랭크 계산
    rank_con = rank(controllability_matrix);
debug_info.rank = rank_con;

    n = length(A);

 

    if rank_con < n || any(del_umax < abs(del_uc))
        FCM = 0;
    else
        FCM = 1;
    end

if FCM == 0
    fprintf('\n--- FCM=0 DETECTED (Clock: %f) ---\n', debug_info.clock);
    disp('Initial A Matrix:');
    disp(debug_info.A);
    disp('Initial B Matrix:');
    disp(debug_info.B_initial);
    disp('ER (for M calculation):');
    disp(debug_info.ER)

      disp('corrcoef_result:');
    disp(debug_info.corrcoef_result)
    
    disp('Calculated M Matrix:');
    disp(debug_info.M);
    disp('Updated B Matrix (B*M):');
    disp(debug_info.B_updated);
    disp('Final Error (for del_uc):');
    disp(debug_info.err_final);
    disp('Required Control |del_uc|:');
    disp(debug_info.del_uc_abs);
    disp('Max Available Control |del_umax|:');
    disp(debug_info.del_umax);
    disp('Controllability Matrix Rank:');
    disp(debug_info.rank);
    fprintf('-------------------------------------\n\n');
end



    [FCMW_, avg_array_FCM_] = calculate_FCMW(FCM,window_size_);

    FCMW = FCMW_;
    avg_array_FCM = avg_array_FCM_;



    if sqrt((x-target_x)^2 + (y-target_y)^2 + (z-target_z)^2) < 10
        FCM_saturated = FCM;
    else
        FCM_saturated = 0;
    end

    [FCMW_saturated_, avg_array_FCM_saturated_] = calculate_FCMW_saturated(FCM_saturated,window_size_);

    FCMW_saturated = FCMW_saturated_;
    avg_array_FCM_saturated = avg_array_FCM_saturated_;


end % if end

disp('-----------------');

end

== matlab function data_collection/MATLAB Function10 ==
  data: xyz_error input; y output
function y = two_norm(xyz_error)
    coder.extrinsic('norm'); % MATLAB 함수 사용을 알림
    
    

    
    % 'y'를 명확히 초기화
    y = 0; 
    
y = norm(xyz_error,2);
